simulink model "compute_jacobian"  (R2018a)
settings: Solver=VariableStepAuto  StartTime=0.0  StopTime=10.0  RelTol=1e-3
settings Model: Creator=DEHAEZE  LastModifiedBy=tdehaeze
settings DataIOCC: SaveOutput=off  SaveTime=off

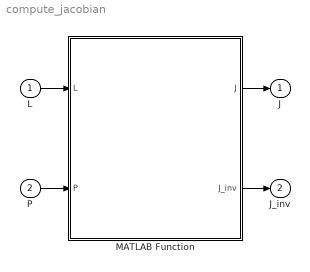
== system compute_jacobian ==
  L : Inport  OutDataTypeStr=double  PortDimensions=[3 6]  SampleTime=0
  P : Inport  Port=2  OutDataTypeStr=double  PortDimensions=[3 6]  SampleTime=0
  MATLAB Function : MATLAB Function  TreatAsAtomicUnit=on
  J : Outport  OutDataTypeStr=double  PortDimensions=[6 6]  SampleTime=0
  J_inv : Outport  Port=2  OutDataTypeStr=double  PortDimensions=[6 6]  SampleTime=0
  wires:
  L/1 -> MATLAB Function/1(L)
  P/1 -> MATLAB Function/2(P)
  MATLAB Function/1(J) -> J/1
  MATLAB Function/2(J_inv) -> J_inv/1

== matlab function compute_jacobian/MATLAB Function ==
  data: L input; J output; P input; J_inv output
function [J, J_inv]  = computeJacobian(L,P)
    J = zeros(6);
    J(:, 1:3) = L';
    J(:, 4:6) = cross(P, L)';
    J_inv = pinv(J);
end
